simulink model "Ex21"  (R2021a)
settings: Solver=VariableStepAuto  StartTime=0.0  StopTime=10  RelTol=1e-3
undefined symbols (not defined in the file): D, FB, g, I, M, tau_B
libraries: vrlib x1
settings Model: Creator=Hans Kristian  LastModifiedBy=olivernorborg
settings SolverCC: AlgebraicLoopSolver=TrustRegion
settings DebuggingCC: SFMachineParentedDataDiag=warning

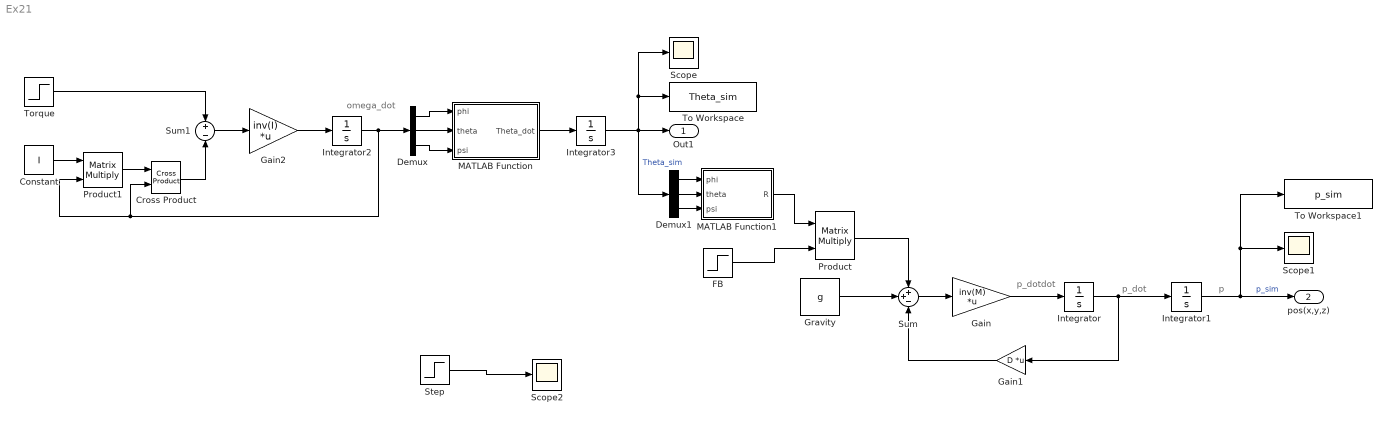
== system Ex21 ==
  note: omega_dot
  note: p_dotdot
  note: p_dot
  note: p
  Constant : Constant  Value=I
  Cross Product : vrlib/Utilities/Cross Product
  Demux : Demux  Outputs=3
  Demux1 : Demux  Outputs=3
  FB : Step  After=FB  SampleTime=0
  Gain : Gain  Gain=inv(M)  Multiplication=Matrix(K*u)
  Gain1 : Gain  Gain=D  Multiplication=Matrix(K*u)
  Gain2 : Gain  Gain=inv(I)  Multiplication=Matrix(K*u)
  Gravity : Constant  Value=g
  Integrator{,1..3} (4 alike) : Integrator
  MATLAB Function : MATLAB Function  TreatAsAtomicUnit=on
  MATLAB Function1 : MATLAB Function  TreatAsAtomicUnit=on
  Product : Product  Multiplication=Matrix(*)
  Product1 : Product  Multiplication=Matrix(*)
  Scope : Scope
  Scope1 : Scope
  Scope2 : Scope
  Step : Step  Time=2  Before=1  After=0  SampleTime=4
  Sum : Sum  Inputs=++-
  Sum1 : Sum  Inputs=+|-
  To Workspace : ToWorkspace  VariableName=Theta_sim  SaveFormat=Timeseries  SampleTime=-1
      settings: Decimation=2
  To Workspace1 : ToWorkspace  VariableName=p_sim  SaveFormat=Timeseries  SampleTime=-1
      settings: Decimation=2
  Torque : Step  After=tau_B  SampleTime=0
  Out1 : Outport  SignalName=Theta_sim
  pos(x,y,z) : Outport  Port=2  SignalName=p
  wires:
  Gravity/1 -> Sum/2
  Product/1 -> Sum/1
  Sum/1 -> Gain/1
  Gain/1 -> Integrator/1
  Integrator/1 -> Gain1/1, Integrator1/1
  Gain1/1 -> Sum/3
  Integrator1/1 -> To Workspace1/1, Scope1/1, pos(x,y,z)/1  "p_sim"
  Torque/1 -> Sum1/1
  Cross Product/1 -> Sum1/2
  Constant/1 -> Product1/1
  Product1/1 -> Cross Product/1
  Gain2/1 -> Integrator2/1
  Demux/1 -> MATLAB Function/1(phi)
  Demux/2 -> MATLAB Function/2(theta)
  Demux/3 -> MATLAB Function/3(psi)
  MATLAB Function/1(Theta_dot) -> Integrator3/1
  Integrator3/1 -> Out1/1, To Workspace/1, Scope/1, Demux1/1  "Theta_sim"
  MATLAB Function1/1(R) -> Product/1
  Demux1/1 -> MATLAB Function1/1(phi)
  Demux1/2 -> MATLAB Function1/2(theta)
  Demux1/3 -> MATLAB Function1/3(psi)
  Sum1/1 -> Gain2/1
  Integrator2/1 -> Cross Product/2, Product1/2, Demux/1
  FB/1 -> Product/2
  Step/1 -> Scope2/1

== matlab function Ex21/MATLAB Function ==
  data: phi input; Theta_dot output; theta input; psi input
function Theta_dot = Theta_dot(phi,theta,psi)
    rot =  [1, 0, -sin(theta);
        0, cos(phi), cos(theta)*sin(phi);
        0, -sin(phi), cos(theta)*cos(phi)
       ];
   omega = [phi;theta;psi];
Theta_dot = inv(rot)*omega;

== matlab function Ex21/MATLAB Function1 ==
  data: phi input; R output; theta input; psi input
function R = Rot(phi,theta,psi)
    Rot = [cos(psi)*cos(theta), -sin(psi)*cos(phi) + cos(psi)*sin(theta)*sin(phi), sin(psi)*sin(phi) + cos(psi)*sin(theta)*cos(phi);
     sin(psi)*cos(theta), cos(psi)*cos(phi) + sin(psi)*sin(theta)*sin(phi), -cos(psi)*sin(phi) + sin(psi)*sin(theta)*cos(phi);
     -sin(theta), cos(theta)*sin(phi), cos(theta)*cos(phi)
    ];
R = Rot;
